simulink model "scheme_3A3"  (R2021b)
settings: Solver=VariableStepAuto  StartTime=0.0  StopTime=500.0  RelTol=1e-3
model workspace (MAT data in the model file):
  Ti = 200
settings Model: Creator=valeria  LastModifiedBy=Ivan
settings SolverCC: AlgebraicLoopSolver=TrustRegion
settings DataIOCC: ReturnWorkspaceOutputsName=out3
settings DebuggingCC: SFMachineParentedDataDiag=warning

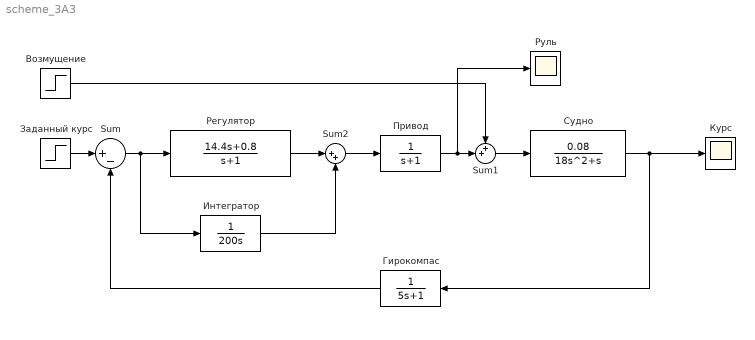
== system scheme_3A3 ==
  " Гирокомпас" : TransferFcn  Denominator=[5 1]
  " Интегратор" : TransferFcn  Denominator=[200 0]
  Sum : Sum  Inputs=|+-
  Sum1 : Sum  Inputs=++|
  Sum2 : Sum  Inputs=|++
  Возмущение : Step  Time=0  After=2  SampleTime=0
  Заданный курс : Step  Time=0  After=10  SampleTime=0
  Курс : Scope
  Привод : TransferFcn  Denominator=[1 1]
  Регулятор : TransferFcn  Numerator=[14.4 0.8]  Denominator=[1 1]
  Руль : Scope
  Судно : TransferFcn  Numerator=[0.08]  Denominator=[18 1 0]
  wires:
  Заданный курс/1 -> Sum/1
  Sum/1 -> " Интегратор"/1, Регулятор/1
  Судно/1 -> Курс/1, " Гирокомпас"/1
  " Гирокомпас"/1 -> Sum/2
  Sum1/1 -> Судно/1
  Привод/1 -> Руль/1, Sum1/2
  Возмущение/1 -> Sum1/1
  Регулятор/1 -> Sum2/1
  Sum2/1 -> Привод/1
  " Интегратор"/1 -> Sum2/2
